simulink model "full_sim_ThorneFleissner"  (R2020b)
settings: Solver=VariableStepAuto  StartTime=0.0  StopTime=10.0  RelTol=1e-3
values from neighbouring files (symbols this model uses):
  Map = im2double(Map).*255    [Configuration.m]    (also in ConfigurationCreation.m)
libraries: simulink_extras x4
settings Model: Creator=rthom  LastModifiedBy=rthom

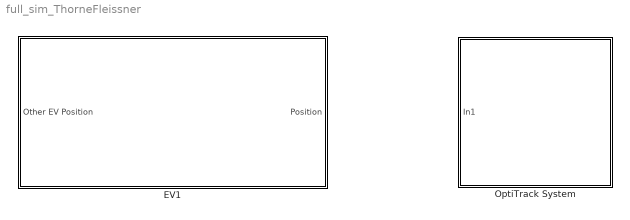
== system full_sim_ThorneFleissner ==
  EV1 : Subsystem
  OptiTrack System : Subsystem

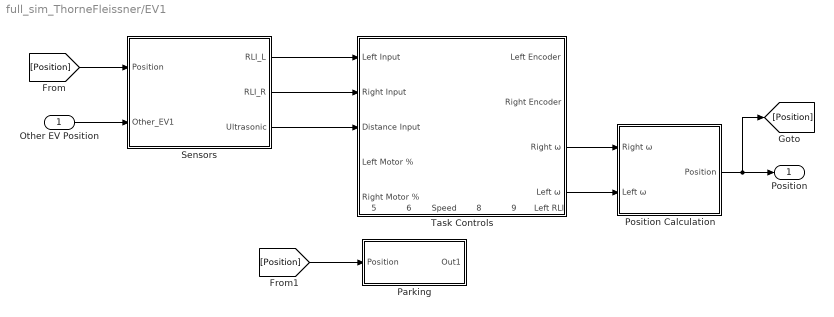
== system full_sim_ThorneFleissner/EV1 ==
  Other EV Position : Inport
  Parking : Subsystem
  Position Calculation : Subsystem
  Sensors : Subsystem
  Task Controls : Subsystem
      settings: PortSchema="{\"entries\":[{\"content\":{\"sides\":[{\"content\":{\"connectorIds\":[\"In1\",\"In2\",\"In3\",\"In4\",\"In5\"]},\"type\":\"ConnectorPlacement.EquallySpacedRectSide\",\"uuid\":\"3c64813c-625d-49d1-ae67-306451c3c1fa\"},{\"content\":{\"connectorIds\":[\"Out1\",\"Out2\",\"Out3\",\"Out4\"],\"side\":\"RIGHT\"},\"type\":\"ConnectorPlacement.EquallySpacedRectSide\",\"uuid\":\"91793cf5-b7a0-4d71-a2c0-83cdd43afca2\"},{\"content\":{\"connectorIds\":[],\"side\":\"TOP\"},\"type\":\"ConnectorPlacement.EquallySpacedRectSide\",\"uuid\":\"5300aefe-28d7-4142-9759-b53f625cf082\"},{\"content\":{\"connectorIds\":[\"Out5\",\"Out6\",\"Out7\",\"Out8\",\"Out9\",\"Out10\"],\"side\":\"BOTTOM\"},\"type\":\"ConnectorPlacement.EquallySpacedRectSide\",\"uuid\":\"7541b0a2-c079-4b1b-9276-8e4ee5949dfd\"},{\"content\":{\"connectorIds\":[],\"side\":\"HIDDEN\"},\"type\":\"ConnectorPlacement.EquallySpacedRectSide\",\"uuid\":\"d0ef4c96-52b1-4a81-ac1e-c57b650a37a1\"}]},\"type\":\"ConnectorPlacement.EquallySpacedConnector\",\"uuid\":\"d02aae7f-e4d5-4935-81ce-eef5c5855771\"}],\"packageUris\":[\"http://schema.mathworks.com/mf0/Connector/R2020b\"],\"version\":\"1.0\"}"
  Position : Outport
  wires:
  Position Calculation/1(Position) -> [Position], Position/1
  Task Controls/3(Right ω) -> Position Calculation/1(Right ω)
  Task Controls/4(Left ω) -> Position Calculation/2(Left ω)
  Sensors/3(Ultrasonic) -> Task Controls/3(Distance Input)
  Sensors/1(RLI_L) -> Task Controls/1(Left Input)
  Sensors/2(RLI_R) -> Task Controls/2(Right Input)
  Other EV Position/1 -> Sensors/2(Other_EV1)
  [Position] -> Sensors/1(Position)
  [Position] -> Parking/1(Position)

== system full_sim_ThorneFleissner/OptiTrack System ==
  In1 : Inport

== system full_sim_ThorneFleissner/EV1/Parking ==
  Position : Inport
  Demux : Demux  Outputs=3
  Parking States : Stateflow chart  TreatAsAtomicUnit=on
  Out1 : Outport
  wires:
  Position/1 -> Demux/1
  Demux/1 -> Parking States/1(data)  "x"
  Demux/2 -> Parking States/2(data1)  "y"
  Demux/3 -> Parking States/3(data2)  "theta"

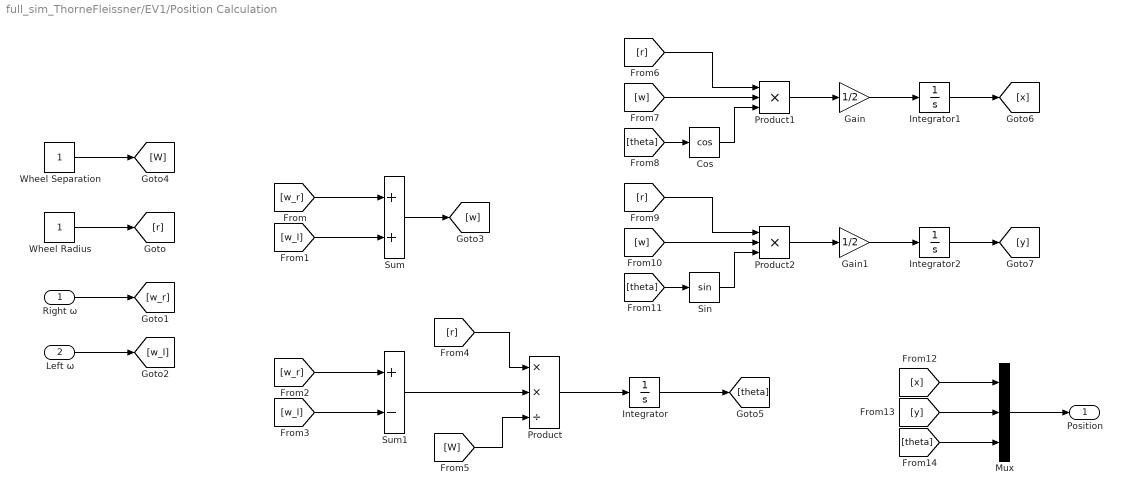
== system full_sim_ThorneFleissner/EV1/Position Calculation ==
  Right ω : Inport
  Left ω : Inport  Port=2
  Cos : Trigonometry  Operator=cos
  Gain : Gain  Gain=1/2
  Gain1 : Gain  Gain=1/2
  Integrator : Integrator
  Integrator1 : Integrator
  Integrator2 : Integrator
  Mux : Mux  Inputs=3
  Product : Product  Inputs=**/
  Product1 : Product  Inputs=3
  Product2 : Product  Inputs=3
  Sin : Trigonometry
  Sum : Sum
  Sum1 : Sum  Inputs=+-
  Wheel Radius : Constant
  Wheel Separation : Constant
  Position : Outport
  wires:
  Wheel Radius/1 -> [r]
  Right ω/1 -> [w_r]
  Left ω/1 -> [w_l]
  [w_r] -> Sum/1
  [w_l] -> Sum/2
  Sum/1 -> [w]
  [w_l] -> Sum1/2
  [w_r] -> Sum1/1
  [r] -> Product/1
  Sum1/1 -> Product/2
  Wheel Separation/1 -> [W]
  [W] -> Product/3
  Product/1 -> Integrator/1
  Integrator/1 -> [theta]
  [theta] -> Cos/1
  Cos/1 -> Product1/3
  [w] -> Product1/2
  [r] -> Product1/1
  Sin/1 -> Product2/3
  [theta] -> Sin/1
  [w] -> Product2/2
  [r] -> Product2/1
  Product1/1 -> Gain/1
  Product2/1 -> Gain1/1
  Gain1/1 -> Integrator2/1
  Gain/1 -> Integrator1/1
  Integrator2/1 -> [y]
  Integrator1/1 -> [x]
  [x] -> Mux/1
  [y] -> Mux/2
  [theta] -> Mux/3
  Mux/1 -> Position/1

== system full_sim_ThorneFleissner/EV1/Sensors ==
  Position : Inport
  Other_EV1 : Inport  Port=2
  Light Sensor Simulation : Subsystem
  Ultrasonic System Simulation : Subsystem
  RLI_L : Outport
  RLI_R : Outport  Port=2
  Ultrasonic : Outport  Port=3
  wires:
  Ultrasonic System Simulation/1(ultrasonic) -> Ultrasonic/1
  Position/1 -> Light Sensor Simulation/1(Position), Ultrasonic System Simulation/1(Position)
  Light Sensor Simulation/1(RLI_R) -> RLI_R/1
  Light Sensor Simulation/2(RLI_L) -> RLI_L/1
  Other_EV1/1 -> Ultrasonic System Simulation/2(Other Position)

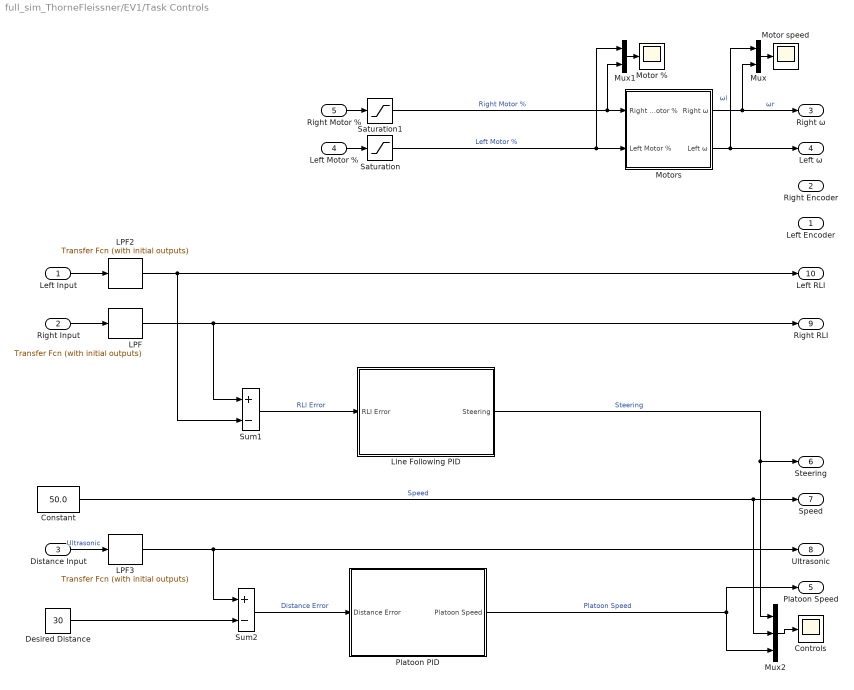
== system full_sim_ThorneFleissner/EV1/Task Controls ==
  Left Input : Inport
  Right Input : Inport  Port=2
  Distance Input : Inport  Port=3
  Left Motor % : Inport  Port=4
  Right Motor % : Inport  Port=5
  Constant : Constant  Value=50.0
  Controls : Scope
  Desired Distance : Constant  Value=30
  LPF : simulink_extras/Additional Linear/Transfer Fcn (with initial outputs)  N=[1]  D="[0.02  1]"  Y0=0  U0=0
  LPF2 : simulink_extras/Additional Linear/Transfer Fcn (with initial outputs)  N=[1]  D="[0.02  1]"  Y0=0  U0=0
  LPF3 : simulink_extras/Additional Linear/Transfer Fcn (with initial outputs)  N=[1]  D="[0.02  1]"  Y0=0  U0=0
  Line Following PID : Subsystem
  Motor % : Scope
  Motor speed : Scope
  Motors : Subsystem
  Mux : Mux  Inputs=2
  Mux1 : Mux  Inputs=2
  Mux2 : Mux  Inputs=3
  Platoon PID : Subsystem
  Saturation : Saturate  UpperLimit=100  LowerLimit=-100
  Saturation1 : Saturate  UpperLimit=100  LowerLimit=-100
  Sum1 : Sum  Inputs=+-
  Sum2 : Sum  Inputs=+-
  Left Encoder : Outport
  Right Encoder : Outport  Port=2
  Right ω : Outport  Port=3
  Left ω : Outport  Port=4
  Platoon Speed : Outport  Port=5
  Steering : Outport  Port=6
  Speed : Outport  Port=7
  Ultrasonic : Outport  Port=8
  Right RLI : Outport  Port=9
  Left RLI : Outport  Port=10
  wires:
  LPF2/1 -> Sum1/2, Left RLI/1
  Motors/1(Right ω) -> Mux/2, Right ω/1  "ωr"
  Motors/2(Left ω) -> Mux/1, Left ω/1  "ωl"
  Mux/1 -> Motor speed/1
  Mux1/1 -> Motor %/1
  Saturation1/1 -> Motors/1(Right Motor %), Mux1/2  "Right Motor %"
  Saturation/1 -> Motors/2(Left Motor %), Mux1/1  "Left Motor %"
  Constant/1 -> Mux2/2, Speed/1  "Speed"
  Left Motor %/1 -> Saturation/1
  Right Motor %/1 -> Saturation1/1
  Mux2/1 -> Controls/1
  Right Input/1 -> LPF/1
  LPF/1 -> Sum1/1, Right RLI/1
  Left Input/1 -> LPF2/1
  Distance Input/1 -> LPF3/1  "Ultrasonic"
  Desired Distance/1 -> Sum2/2
  LPF3/1 -> Sum2/1, Ultrasonic/1
  Platoon PID/1(Platoon Speed) -> Mux2/3, Platoon Speed/1  "Platoon Speed"
  Sum2/1 -> Platoon PID/1(Distance Error)  "Distance Error"
  Line Following PID/1(Steering) -> Mux2/1, Steering/1  "Steering"
  Sum1/1 -> Line Following PID/1(RLI Error)  "RLI Error"

== system full_sim_ThorneFleissner/EV1/Sensors/Light Sensor Simulation ==
  Position : Inport
  Create Position : MATLAB Function  TreatAsAtomicUnit=on
  Map : Constant  Value=Map
  Radius : Constant  Value=22
  RLI_R : Outport
  RLI_L : Outport  Port=2
  wires:
  Position/1 -> Create Position/1(Position)
  Map/1 -> Create Position/2(Map)
  Radius/1 -> Create Position/3(Radius)
  Create Position/2(RLI_L) -> RLI_L/1
  Create Position/1(RLI_R) -> RLI_R/1

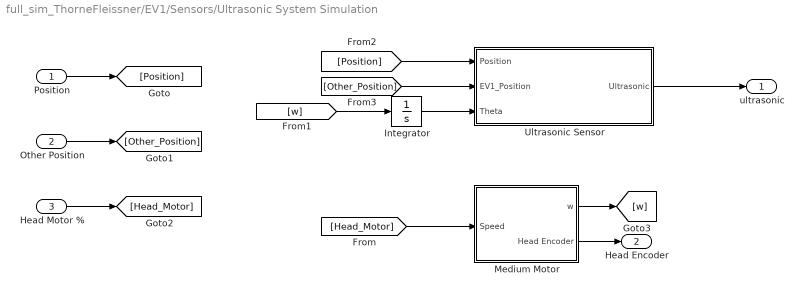
== system full_sim_ThorneFleissner/EV1/Sensors/Ultrasonic System Simulation ==
  Position : Inport
  Other Position : Inport  Port=2
  Head Motor % : Inport  Port=3
  Integrator : Integrator
  Medium Motor : Subsystem
  Ultrasonic Sensor : MATLAB Function  TreatAsAtomicUnit=on
  ultrasonic : Outport
  Head Encoder : Outport  Port=2
  wires:
  Position/1 -> [Position]
  Head Motor %/1 -> [Head_Motor]
  Other Position/1 -> [Other_Position]
  [Head_Motor] -> Medium Motor/1(Speed)
  Ultrasonic Sensor/1(Ultrasonic) -> ultrasonic/1
  Medium Motor/1(w) -> [w]
  Medium Motor/2(Head Encoder) -> Head Encoder/1
  [Other_Position] -> Ultrasonic Sensor/2(EV1_Position)
  [Position] -> Ultrasonic Sensor/1(Position)
  [w] -> Integrator/1
  Integrator/1 -> Ultrasonic Sensor/3(Theta)

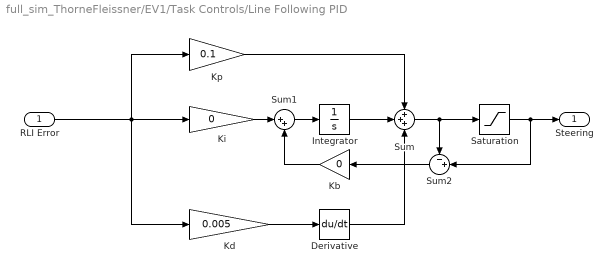
== system full_sim_ThorneFleissner/EV1/Task Controls/Line Following PID ==
  RLI Error : Inport
  Derivative : Derivative
  Integrator : Integrator
  Kb : Gain  Gain=0
  Kd : Gain  Gain=0.005
  Ki : Gain  Gain=0
  Kp : Gain  Gain=0.1
  Saturation : Saturate  UpperLimit=15  LowerLimit=-15
  Sum : Sum  Inputs=+++
  Sum1 : Sum  Inputs=|++
  Sum2 : Sum  Inputs=-+|
  Steering : Outport
  wires:
  Sum/1 -> Sum2/1, Saturation/1
  Kd/1 -> Derivative/1
  Kp/1 -> Sum/1
  Integrator/1 -> Sum/2
  RLI Error/1 -> Kd/1, Ki/1, Kp/1
  Derivative/1 -> Sum/3
  Saturation/1 -> Sum2/2, Steering/1
  Ki/1 -> Sum1/1
  Sum1/1 -> Integrator/1
  Kb/1 -> Sum1/2
  Sum2/1 -> Kb/1

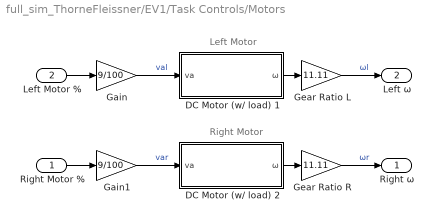
== system full_sim_ThorneFleissner/EV1/Task Controls/Motors ==
  note: Left Motor
  note: Right Motor
  Right Motor % : Inport
  Left Motor % : Inport  Port=2
  DC Motor (w/ load) 1 : Subsystem
  DC Motor (w/ load) 2 : Subsystem
  Gain : Gain  Gain=9/100
  Gain1 : Gain  Gain=9/100
  Gear Ratio L : Gain  Gain=11.11
  Gear Ratio R : Gain  Gain=11.11
  Right ω : Outport
  Left ω : Outport  Port=2
  wires:
  DC Motor (w/ load) 1/1(ω) -> Gear Ratio L/1
  Right Motor %/1 -> Gain1/1
  Gear Ratio L/1 -> Left ω/1  "ωl"
  DC Motor (w/ load) 2/1(ω) -> Gear Ratio R/1
  Left Motor %/1 -> Gain/1
  Gain/1 -> DC Motor (w/ load) 1/1(va)  "val"
  Gear Ratio R/1 -> Right ω/1  "ωr"
  Gain1/1 -> DC Motor (w/ load) 2/1(va)  "var"

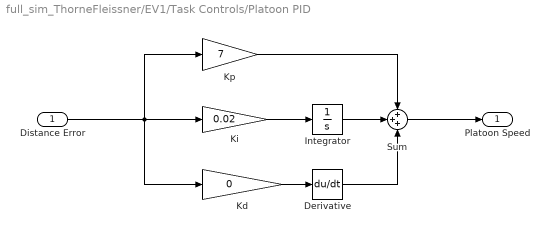
== system full_sim_ThorneFleissner/EV1/Task Controls/Platoon PID ==
  Distance Error : Inport
  Derivative : Derivative
  Integrator : Integrator
  Kd : Gain  Gain=0
  Ki : Gain  Gain=0.02
  Kp : Gain  Gain=7
  Sum : Sum  Inputs=+++
  Platoon Speed : Outport
  wires:
  Sum/1 -> Platoon Speed/1
  Kd/1 -> Derivative/1
  Kp/1 -> Sum/1
  Ki/1 -> Integrator/1
  Integrator/1 -> Sum/2
  Distance Error/1 -> Kd/1, Ki/1, Kp/1
  Derivative/1 -> Sum/3

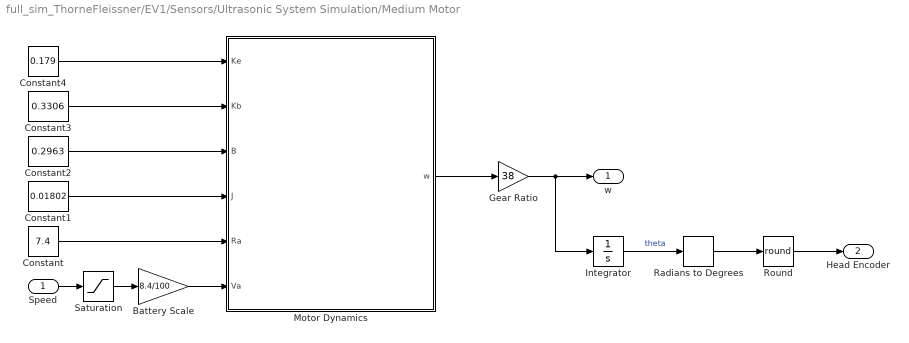
== system full_sim_ThorneFleissner/EV1/Sensors/Ultrasonic System Simulation/Medium Motor ==
  Speed : Inport
  Battery Scale : Gain  Gain=8.4/100
  Constant : Constant  Value=7.4
  Constant1 : Constant  Value=0.01802
  Constant2 : Constant  Value=0.2963
  Constant3 : Constant  Value=0.3306
  Constant4 : Constant  Value=0.179
  Gear Ratio : Gain  Gain=38
  Integrator : Integrator
  Motor Dynamics : Subsystem
  Radians to Degrees : simulink_extras/Transformations/Radians to Degrees
  Round : Rounding  Operator=round
  Saturation : Saturate  UpperLimit=100  LowerLimit=-100
  w : Outport
  Head Encoder : Outport  Port=2
  wires:
  Constant/1 -> Motor Dynamics/5(Ra)
  Constant1/1 -> Motor Dynamics/4(J)
  Constant2/1 -> Motor Dynamics/3(B)
  Constant3/1 -> Motor Dynamics/2(Kb)
  Constant4/1 -> Motor Dynamics/1(Ke)
  Motor Dynamics/1(w) -> Gear Ratio/1
  Gear Ratio/1 -> Integrator/1, w/1
  Battery Scale/1 -> Motor Dynamics/6(Va)
  Speed/1 -> Saturation/1
  Saturation/1 -> Battery Scale/1
  Integrator/1 -> Radians to Degrees/1  "theta"
  Radians to Degrees/1 -> Round/1
  Round/1 -> Head Encoder/1

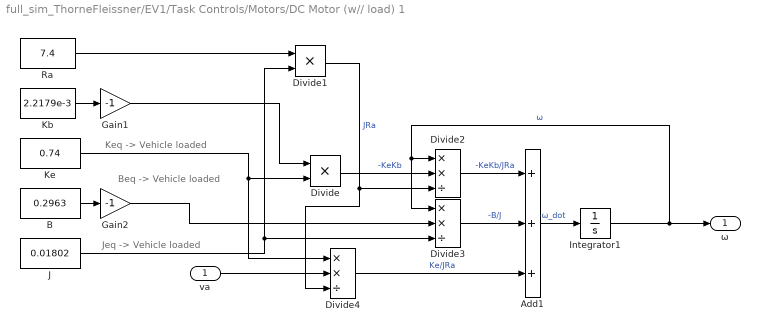
== system full_sim_ThorneFleissner/EV1/Task Controls/Motors/DC Motor (w// load) 1 ==
  note: Keq -> Vehicle loaded
  note: Jeq -> Vehicle loaded
  note: Beq -> Vehicle loaded
  va : Inport
  Add1 : Sum  Inputs=+++
  B : Constant  Value=0.2963
  Divide : Product  Inputs=**
  Divide1 : Product  Inputs=**
  Divide2 : Product  Inputs=**/
  Divide3 : Product  Inputs=**/
  Divide4 : Product  Inputs=**/
  Gain1 : Gain  Gain=-1
  Gain2 : Gain  Gain=-1
  Integrator1 : Integrator
  J : Constant  Value=0.01802
  Kb : Constant  Value=2.2179e-3
  Ke : Constant  Value=0.74
  Ra : Constant  Value=7.4
  ω : Outport
  wires:
  Divide2/1 -> Add1/1  "-KeKb/JRa"
  Divide3/1 -> Add1/2  "-B/J"
  Ra/1 -> Divide1/1
  Kb/1 -> Gain1/1
  Ke/1 -> Divide4/1, Divide/2
  J/1 -> Divide1/2, Divide3/3
  B/1 -> Gain2/1
  Gain2/1 -> Divide3/2
  Add1/1 -> Integrator1/1  "ω_dot"
  va/1 -> Divide4/2
  Gain1/1 -> Divide/1
  Divide/1 -> Divide2/2  "-KeKb"
  Divide1/1 -> Divide2/3, Divide4/3  "JRa"
  Divide4/1 -> Add1/3  "Ke/JRa"
  Integrator1/1 -> Divide3/1, Divide2/1, ω/1  "ω"

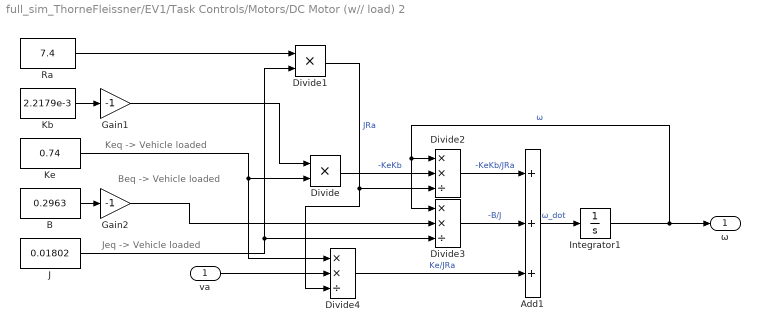
== system full_sim_ThorneFleissner/EV1/Task Controls/Motors/DC Motor (w// load) 2 ==
  note: Keq -> Vehicle loaded
  note: Jeq -> Vehicle loaded
  note: Beq -> Vehicle loaded
  va : Inport
  Add1 : Sum  Inputs=+++
  B : Constant  Value=0.2963
  Divide : Product  Inputs=**
  Divide1 : Product  Inputs=**
  Divide2 : Product  Inputs=**/
  Divide3 : Product  Inputs=**/
  Divide4 : Product  Inputs=**/
  Gain1 : Gain  Gain=-1
  Gain2 : Gain  Gain=-1
  Integrator1 : Integrator
  J : Constant  Value=0.01802
  Kb : Constant  Value=2.2179e-3
  Ke : Constant  Value=0.74
  Ra : Constant  Value=7.4
  ω : Outport
  wires:
  Divide2/1 -> Add1/1  "-KeKb/JRa"
  Divide3/1 -> Add1/2  "-B/J"
  Ra/1 -> Divide1/1
  Kb/1 -> Gain1/1
  Ke/1 -> Divide4/1, Divide/2
  J/1 -> Divide1/2, Divide3/3
  B/1 -> Gain2/1
  Gain2/1 -> Divide3/2
  Add1/1 -> Integrator1/1  "ω_dot"
  va/1 -> Divide4/2
  Gain1/1 -> Divide/1
  Divide/1 -> Divide2/2  "-KeKb"
  Divide1/1 -> Divide2/3, Divide4/3  "JRa"
  Divide4/1 -> Add1/3  "Ke/JRa"
  Integrator1/1 -> Divide3/1, Divide2/1, ω/1  "ω"

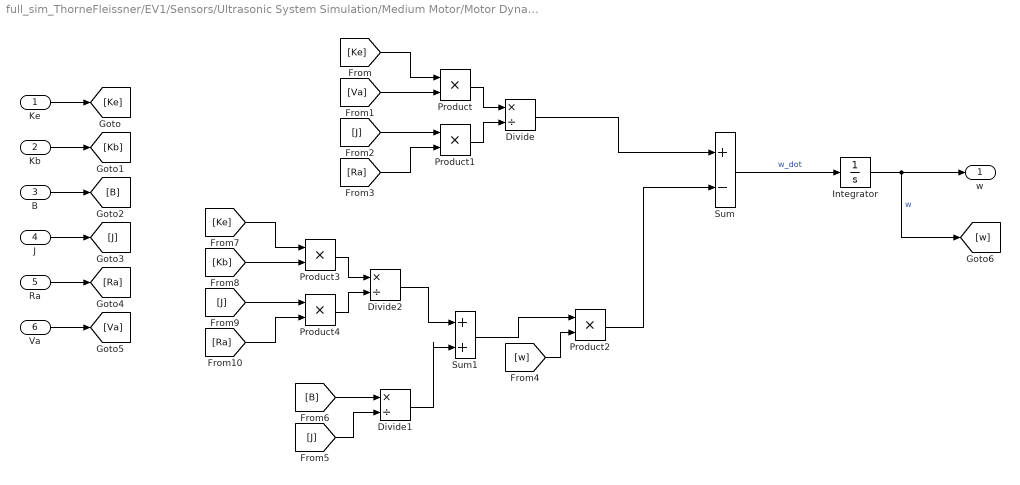
== system full_sim_ThorneFleissner/EV1/Sensors/Ultrasonic System Simulation/Medium Motor/Motor Dynamics ==
  Ke : Inport
  Kb : Inport  Port=2
  B : Inport  Port=3
  J : Inport  Port=4
  Ra : Inport  Port=5
  Va : Inport  Port=6
  Divide : Product  Inputs=*/
  Divide1 : Product  Inputs=*/
  Divide2 : Product  Inputs=*/
  Integrator : Integrator
  Product{,1..4} (5 alike) : Product
  Sum : Sum  Inputs=+-
  Sum1 : Sum
  w : Outport
  wires:
  Integrator/1 -> [w], w/1  "w"
  Sum/1 -> Integrator/1  "w_dot"
  Ke/1 -> [Ke]
  Kb/1 -> [Kb]
  B/1 -> [B]
  J/1 -> [J]
  Ra/1 -> [Ra]
  Va/1 -> [Va]
  Product/1 -> Divide/1
  Product1/1 -> Divide/2
  [Ke] -> Product/1
  [Va] -> Product/2
  [J] -> Product1/1
  [Ra] -> Product1/2
  Divide/1 -> Sum/1
  Product2/1 -> Sum/2
  [w] -> Product2/2
  Sum1/1 -> Product2/1
  Divide1/1 -> Sum1/2
  [J] -> Divide1/2
  [B] -> Divide1/1
  [Ra] -> Product4/2
  Product3/1 -> Divide2/1
  Product4/1 -> Divide2/2
  [J] -> Product4/1
  [Ke] -> Product3/1
  [Kb] -> Product3/2
  Divide2/1 -> Sum1/1

== matlab function full_sim_ThorneFleissner/EV1/Sensors/Light Sensor Simulation/Create Position ==
  data: Position input; Map input; Radius input; RLI_R output; RLI_L output
function [RLI_R,RLI_L] = CreatePosition(Position,Map,Radius)
%Position of Light Sensors (based on EV Center of Mass)
    x = Position(1) + 0.6*cos(Position(3));%Calculate x position of front of vehicle
    y = Position(2) + 0.6*sin(Position(3));%Calculate y position of front of vehicle

    %Need to change so that bottom left is 0,0. Need to find what top value
    %is in m and pixels.
    TopOptiTrack = 2.936;%m, top boundary of map from OptiTrack
    LeftOptiTrack = -1.9;%m, left boundary of map from OptiTrack

    TopPixel = 69;%pixel, top boundary of map from image
    LeftPixel = 71;%pixel, left boundary of map from image

    xScale = 144.4175;%Scale factor between pixels and real values from OptiTrack for x
    yScale = -140.7979;%Scale factor between pixels and real values from OptiTrack for y

    x_Pixel = LeftPixel + (xScale*(x - LeftOptiTrack));%Convert the x position of front of vehicle into pixels
    y_Pixel = TopPixel + (yScale*(y - TopOptiTrack));%Convert the y position of front of vehicle into pixels


    x_LeftSensor = x_Pixel - 34*sin(Position(3));%Calculate Left Sensor x Position in pixels
    y_LeftSensor = y_Pixel - 34*cos(Position(3));%Calculate Left Sensor y Position in pixels

    x_RightSensor = x_Pixel + 34*sin(Position(3));%Calculate Right Sensor x Position in pixels
    y_RightSensor = y_Pixel + 34*cos(Position(3));%Calculate Right Sensor y Position in pixels
%RLI Shared Code
    X = -Radius:Radius;%Define size of circle in x direction
    Y = -Radius:Radius;%Define size of circle in y direction
    [MX,MY] = meshgrid(X,Y);%Create meshgrid (square) the size of the radius
    
    Circle = MX.^2 + MY.^2 <= Radius^2;%Create mask in shape of circle using meshgrid values
%Right RLI
    X_Boundary_R = x_RightSensor - Radius:x_RightSensor + Radius;%Calculate x coordinate boundary of the light sensor
    Y_Boundary_R = y_RightSensor - Radius:y_RightSensor + Radius;%Calculate y coordinate boundary of the light sensor

    Area_R = Map(Y_Boundary_R,X_Boundary_R);%Define area within the map. Indexing is Map(y,x)
    
    RLI_R = sum(Area_R.*Circle,'all') / sum(Circle,'all');%Calculate the average of values over the circular area;
%     RLI_R = round(RLI_R*.7 + 10);%I don't know what this is for yet. 

%Left RLI
    X_Boundary_L = x_LeftSensor - Radius:x_LeftSensor + Radius;%Calculate x coordinate boundary of the light sensor
    Y_Boundary_L = y_LeftSensor - Radius:y_LeftSensor + Radius;%Calculate y coordinate boundary of the light sensor

    Area_L = Map(Y_Boundary_L,X_Boundary_L);%Define area within the map. Indexing is Map(y,x)
    
    RLI_L = sum(Area_L.*Circle,'all') / sum(Circle,'all');%Calculate the average of values over the circular area;
%     RLI_L = round(RLI_L*.7 + 10);%I don't know what this is for yet.
end

== stateflow chart full_sim_ThorneFleissner/EV1/Parking/Parking States ==
  data: data input; data1 input; data2 input

== matlab function full_sim_ThorneFleissner/EV1/Sensors/Ultrasonic System Simulation/Ultrasonic Sensor ==
  data: Position input; Ultrasonic output; EV1_Position input; Theta input
function Ultrasonic = UltrasonicFcn(Position,EV1_Position,Theta)
%% Parking Spot Position Constants
    Spot1_Up = [-1.308; 0.9163];
    Spot1_Down = [-1.3115; 0.6954];
    Spot2_Up = [-1.1672; 1.3082];
    Spot2_Down = [-1.1647; 1.0837];
    Spot3_Up = [-0.8906; 1.72];
    Spot3_Down = [-0.8977; 1.5883];

    Spot1_Mid = (Spot1_Up(1:2)+ Spot1_Down(1:2))/2;
    Spot2_Mid = (Spot2_Up(1:2)+ Spot2_Down(1:2))/2;
    Spot3_Mid = (Spot3_Up(1:2)+ Spot3_Down(1:2))/2;

%% Other EV 1
    %Calculate the position between the objects
        EV1_Distance_XZ = EV1_Position(1:2) - Position(1:2);%Calculating the x and z values for the distance between the EV's
        EV1_Distance_Hypot = sqrt((EV1_Distance_XZ(1)^2)+(EV1_Distance_XZ(2)^2));%Calculating hypotenuse using calculated x and z values
        EV1_Distance_Hypot = (EV1_Distance_Hypot*100) - 14;%Convert from m to cm and move points from center of EVs to back of other EV (7cm) and front of EV (7cm) NOTE: 7cm is from center of brick to front of brick, shouldn't it be to the front of the sensor?
    
    %Adjust Boundary of Sensor based on Distance
       
        EV1_Base_Boundary = 10;%Define the base boundary value
        
        if EV1_Distance_Hypot <= 60 && EV1_Distance_Hypot >= 30
          EV1_Boundary = EV1_Base_Boundary + 10; 
        elseif EV1_Distance_Hypot<=30 && EV1_Distance_Hypot>=20
          EV1_Boundary = EV1_Base_Boundary + 20; 
        elseif EV1_Distance_Hypot<20
          EV1_Boundary = EV1_Base_Boundary + 30; 
        end
        
    %Calculate Desired Angle of Ultrasonic Sensor
        EV1_alpha_rad = atan2(EV1_Distance_XZ(2),EV1_Distance_XZ(1)) - Position(3);%Radians, Calculating the desired head angle of the ultrasonic sensor in relation to the EV body
        EV1_alpha_deg = rad2deg(EV1_alpha_rad);%Convert alpha from radians to degrees
        EV1_alpha_desired = mod(EV1_alpha_deg + 180, 360) - 180;%Limit the desired head angle betweeen -180 and 180 deg
        
    %Range Boundary Calculations
        EV1_boundary_pos = EV1_alpha_desired + EV1_Boundary;%Calculate positive boundary
        EV1_boundary_pos = mod(EV1_boundary_pos + 180, 360) - 180;%Limit boundary between -180 and 180
        EV1_boundary_neg = EV1_alpha_desired - EV1_Boundary;%Calculate negative boundary
        EV1_boundary_neg = mod(EV1_boundary_neg + 180, 360) - 180;%Limit boundary between -180 and 180
        
%% Parking Spot 1
    %Calculate the position between the objects
        Spot1_Distance_XZ = Spot1_Mid(1:2) - Position(1:2);%Calculating the x and z values for the distance between the EV and parking spot 1
        Spot1_Distance_Hypot = sqrt((Spot1_Distance_XZ(1)^2)+(Spot1_Distance_XZ(2)^2));%Calculating hypotenuse using calculated x and z values
        Spot1_Distance_Hypot = (Spot1_Distance_Hypot*100) - 7;%Convert from m to cm and move distance to front of EV (NOTE: should probably be front of sensor not EV)

     %Adjust Boundary of Sensor based on Distance
       
        Spot1_Base_Boundary = 10;%Define the base boundary value
        
        if Spot1_Distance_Hypot <= 60 && Spot1_Distance_Hypot >= 30
          Spot1_Boundary = Spot1_Base_Boundary + 10; 
        elseif Spot1_Distance_Hypot<=30 && Spot1_Distance_Hypot>=20
          Spot1_Boundary = Spot1_Base_Boundary + 20; 
        elseif Spot1_Distance_Hypot<20
          Spot1_Boundary = Spot1_Base_Boundary + 30; 
        end
        
    %Calculate Desired Angle of Ultrasonic Sensor
        Spot1_alpha_rad = atan2(Spot1_Distance_XZ(2),Spot1_Distance_XZ(1)) - Position(3);%Radians, Calculating the desired head angle of the ultrasonic sensor in relation to the EV body
        Spot1_alpha_deg = rad2deg(Spot1_alpha_rad);%Convert alpha from radians to degrees
        Spot1_alpha_desired = mod(Spot1_alpha_deg + 180, 360) - 180;%Limit the desired head angle betweeen -180 and 180 deg
        
    %Range Boundary Calculations
        Spot1_boundary_pos = Spot1_alpha_desired + Spot1_Boundary;%Calculate positive boundary
        Spot1_boundary_pos = mod(Spot1_boundary_pos + 180, 360) - 180;%Limit boundary between -180 and 180
        Spot1_boundary_neg = Spot1_alpha_desired - Spot1_Boundary;%Calculate negative boundary
        Spot1_boundary_neg = mod(Spot1_boundary_neg + 180, 360) - 180;%Limit boundary between -180 and 180
        
%% Parking Spot 2
    %Calculate the position between the objects
        Spot2_Distance_XZ = Spot2_Mid(1:2) - Position(1:2);%Calculating the x and z values for the distance between the EV and parking spot 2
        Spot2_Distance_Hypot = sqrt((Spot2_Distance_XZ(1)^2)+(Spot2_Distance_XZ(2)^2));%Calculating hypotenuse using calculated x and z values
        Spot2_Distance_Hypot = (Spot2_Distance_Hypot*100) - 7;%Convert from m to cm and move distance to front of EV (NOTE: should probably be front of sensor not EV)
        
     %Adjust Boundary of Sensor based on Distance
       
        Spot2_Base_Boundary = 10;%Define the base boundary value
        
        if Spot2_Distance_Hypot <= 60 && Spot2_Distance_Hypot >= 30
          Spot2_Boundary = Spot2_Base_Boundary + 10; 
        elseif Spot2_Distance_Hypot<=30 && Spot2_Distance_Hypot>=20
          Spot2_Boundary = Spot2_Base_Boundary + 20; 
        elseif Spot2_Distance_Hypot<20
          Spot2_Boundary = Spot2_Base_Boundary + 30; 
        end
        
    %Calculate Desired Angle of Ultrasonic Sensor
        Spot2_alpha_rad = atan2(Spot2_Distance_XZ(2),Spot2_Distance_XZ(1)) - Position(3);%Radians, Calculating the desired head angle of the ultrasonic sensor in relation to the EV body
        Spot2_alpha_deg = rad2deg(Spot2_alpha_rad);%Convert alpha from radians to degrees
        Spot2_alpha_desired = mod(Spot2_alpha_deg + 180, 360) - 180;%Limit the desired head angle betweeen -180 and 180 deg
        
    %Range Boundary Calculations
        Spot2_boundary_pos = Spot2_alpha_desired + Spot2_Boundary;%Calculate positive boundary
        Spot2_boundary_pos = mod(Spot2_boundary_pos + 180, 360) - 180;%Limit boundary between -180 and 180
        Spot2_boundary_neg = Spot2_alpha_desired - Spot2_Boundary;%Calculate negative boundary
        Spot2_boundary_neg = mod(Spot2_boundary_neg + 180, 360) - 180;%Limit boundary between -180 and 180
        
%% Parking Spot 3
    %Calculate the position between the objects
        Spot3_Distance_XZ = Spot3_Mid(1:2) - Position(1:2);%Calculating the x and z values for the distance between the EV and parking spot 3
        Spot3_Distance_Hypot = sqrt((Spot3_Distance_XZ(1)^2)+(Spot3_Distance_XZ(2)^2));%Calculating hypotenuse using calculated x and z values
        Spot3_Distance_Hypot = (Spot3_Distance_Hypot*100) - 7;%Convert from m to cm and move distance to front of EV (NOTE: should probably be front of sensor not EV)
        
     %Adjust Boundary of Sensor based on Distance
       
        Spot3_Base_Boundary = 10;%Define the base boundary value
        
        if Spot3_Distance_Hypot <= 60 && Spot3_Distance_Hypot >= 30
          Spot3_Boundary = Spot3_Base_Boundary + 10; 
        elseif Spot3_Distance_Hypot<=30 && Spot3_Distance_Hypot>=20
          Spot3_Boundary = Spot3_Base_Boundary + 20; 
        elseif Spot3_Distance_Hypot<20
          Spot3_Boundary = Spot3_Base_Boundary + 30; 
        end
        
    %Calculate Desired Angle of Ultrasonic Sensor
        Spot3_alpha_rad = atan2(Spot3_Distance_XZ(2),Spot3_Distance_XZ(1)) - Position(3);%Radians, Calculating the desired head angle of the ultrasonic sensor in relation to the EV body
        Spot3_alpha_deg = rad2deg(Spot3_alpha_rad);%Convert alpha from radians to degrees
        Spot3_alpha_desired = mod(Spot3_alpha_deg + 180, 360) - 180;%Limit the desired head angle betweeen -180 and 180 deg
        
    %Range Boundary Calculations
        Spot3_boundary_pos = Spot3_alpha_desired + Spot3_Boundary;%Calculate positive boundary
        Spot3_boundary_pos = mod(Spot3_boundary_pos + 180, 360) - 180;%Limit boundary between -180 and 180
        Spot3_boundary_neg = Spot3_alpha_desired - Spot3_Boundary;%Calculate negative boundary
        Spot3_boundary_neg = mod(Spot3_boundary_neg + 180, 360) - 180;%Limit boundary between -180 and 180
        
%% Calculate Ultrasonic Output
    %Calculate Actual Angle of Ultrasonic Sensor
        theta_deg = rad2deg(Theta);%Convert theta from radians to degrees
        theta_actual = mod(theta_deg + 180, 360) - 180;%Limit the actual head angle between -180 and 180 deg
    %Determine Which Distance to Use if within Motor Head Boundary
        Ultrasonic = 255;%cm, Set the default value of the ultrasonic sensor to the maximum output
        
        if (((EV1_boundary_neg <= theta_actual) && (EV1_boundary_pos >= theta_actual)) && (EV1_boundary_pos > EV1_boundary_neg)) ...
            || (~((EV1_boundary_pos <= theta_actual) && (EV1_boundary_neg >= theta_actual)) && (EV1_boundary_neg >= EV1_boundary_pos))
                Ultrasonic = min(Ultrasonic, EV1_Distance_Hypot);
                
        elseif (((Spot1_boundary_neg <= theta_actual) && (Spot1_boundary_pos >= theta_actual)) && (Spot1_boundary_pos > Spot1_boundary_neg)) ...
            || (~((Spot1_boundary_pos <= theta_actual) && (Spot1_boundary_neg >= theta_actual)) && (Spot1_boundary_neg >= Spot1_boundary_pos))
                Ultrasonic = min(Ultrasonic, Spot1_Distance_Hypot);
                
        elseif (((Spot2_boundary_neg <= theta_actual) && (Spot2_boundary_pos >= theta_actual)) && (Spot2_boundary_pos > Spot2_boundary_neg)) ...
            || (~((Spot2_boundary_pos <= theta_actual) && (Spot2_boundary_neg >= theta_actual)) && (Spot2_boundary_neg >= Spot2_boundary_pos))
                Ultrasonic = min(Ultrasonic, Spot2_Distance_Hypot);
                
        elseif (((Spot3_boundary_neg <= theta_actual) && (Spot3_boundary_pos >= theta_actual)) && (Spot3_boundary_pos > Spot3_boundary_neg)) ...
            || (~((Spot3_boundary_pos <= theta_actual) && (Spot3_boundary_neg >= theta_actual)) && (Spot3_boundary_neg >= Spot3_boundary_pos))
                Ultrasonic = min(Ultrasonic, Spot3_Distance_Hypot);
        end
end
